simulink model "day4"  (R2017b)
settings: Solver=VariableStepAuto  StartTime=0.0  StopTime=10.0  RelTol=1e-3
undefined symbols (not defined in the file): X, Y, Z
libraries: simulink x1
settings Model: Creator=Admin  LastModifiedBy=Admin

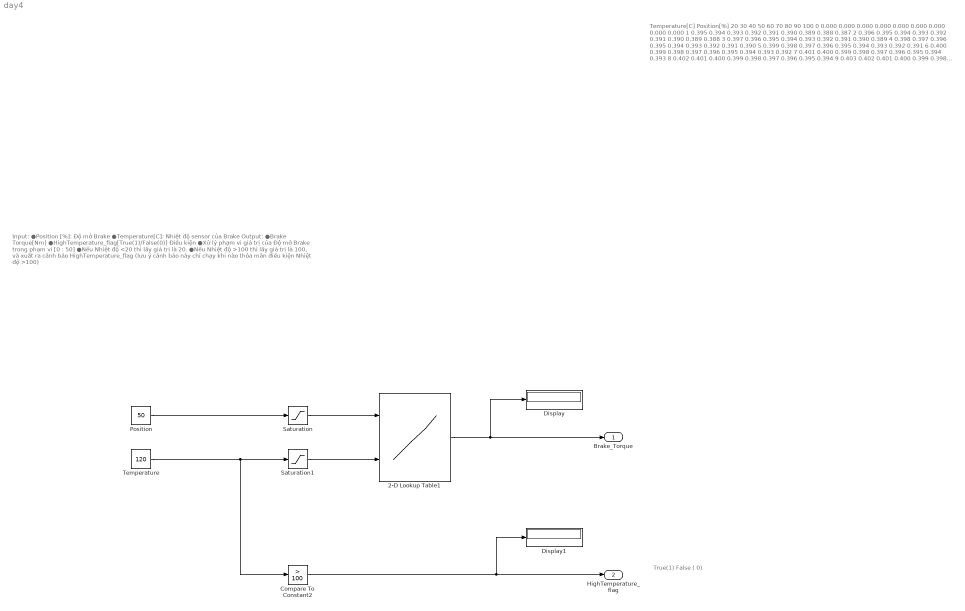
== system day4 ==
  note: Input:
      | ●Position [%]: Độ mở Brake
      | ●Temperature[C]: Nhiệt độ sensor của Brake
      | Output:
      | ●Brake Torque[Nm]
      | ●HighTemperature_flag[True(1)/False(0)]
      | Điều kiện
      | ●Xử lý phạm vi giá trị của Độ mở Brake trong phạm vi [0 : 50]
      | ●Nếu Nhiệt độ <20 thì lấy giá trị là 20.
      | ●Nếu Nhiệt độ >100 thì lấy giá trị là 100, và xuất ra cảnh báo HighTemperature_flag (lưu ý cảnh báo này chỉ chạy khi nào thỏa mãn điều kiện Nhiệt độ >100)
  note: Temperature[C]
      |
      | Position[%]
      | 20
      | 30
      | 40
      | 50
      | 60
      | 70
      | 80
      | 90
      | 100
      |
      | 0
      | 0.000
      | 0.000
      | 0.000
      | 0.000
      | 0.000
      | 0.000
      | 0.000
      | 0.000
      | 0.000
      |
      | 1
      | 0.395
      | 0.394
      | 0.393
      | 0.392
      | 0.391
      | 0.390
      | 0.389
      | 0.388
      | 0.387
      |
      | 2
      | 0.396
      | 0.395
      | 0.394
      | 0.393
      | 0.392
      | 0.391
      | 0.390
      | 0.389
      | 0.388
      |
      | 3
      | 0.397
      | 0.396
      | 0.395
      | 0.394
      | 0.393
      | 0.392
      | 0.391
      | 0.390
      | 0.389
      |
      | 4
      | 0.398
      | 0.397
      | 0.396
      | 0.395
      | 0.394
      | 0.393
      | 0.392
      | 0.391
      | 0.390
      |
      | 5
      | 0.399
      | 0.398
      | 0.397
      | 0.396
      | 0.395
      | 0.394
      | 0.393
      | 0.392
      | 0.391
      |
      | 6
      | 0.400
      | 0.399
      | 0.398
      | 0.397
      | 0.396
      | 0.395
      | 0.394
      | 0.393
      | 0.392
      |
      | 7
      | 0.401
      | 0.400
      | 0.399
      | 0.398
      | 0.397
      | 0.396
      | 0.395
      | 0.394
      | 0.393
      |
      | 8
      | 0.402
      | 0.401
      | 0.400
      | 0.399
      | 0.398
      | 0.397
      | 0.396
      | 0.395
      | 0.394
      |
      | 9
      | 0.403
      | 0.402
      | 0.401
      | 0.400
      | 0.399
      | 0.398
      | 0.397
      | 0.396
      | 0.395
      |
      | 10
      | 0.404
      | 0.403
      | 0.402
      | 0.401
      | 0.400
      | 0.399
      | 0.398
      | 0.397
      | 0.396
      |
      | 11
      | 0.405
      | 0.404
      | 0.403
      | 0.402
      | 0.401
      | 0.400
      | 0.399
      | 0.398
      | 0.397
      |
      | 12
      | 0.406
      | 0.405
      | 0.404
      | 0.403
      | 0.402
      | 0.401
      | 0.400
      | 0.399
      | 0.398
      |
      | 13
      | 0.407
      | 0.406
      | 0.405
      | 0.404
      | 0.403
      | 0.402
      | 0.401
      | 0.400
      | 0.399
      |
      | 14
      | 0.408
      | 0.407
      | 0.406
      | 0.405
      | 0.404
      | 0.403
      | 0.402
      | 0.401
      | 0.400
      |
      | 15
      | 0.409
      | 0.408
      | 0.407
      | 0.406
      | 0.405
      | 0.404
      | 0.403
      | 0.402
      | 0.401
      |
      | 16
      | 0.410
      | 0.409
      | 0.408
      | 0.407
      | 0.406
      | 0.405
      | 0.404
      | 0.403
      | 0.402
      |
      | 17
      | 0.411
      | 0.410
      | 0.409
      | 0.408
      | 0.407
      | 0.406
      | 0.405
      | 0.404
      | 0.403
      |
      | 18
      | 0.412
      | 0.411
      | 0.410
      | 0.409
      | 0.408
      | 0.407
      | 0.406
      | 0.405
      | 0.404
      |
      | 19
      | 0.413
      | 0.412
      | 0.411
      | 0.410
      | 0.409
      | 0.408
      | 0.407
      | 0.406
      | 0.405
      |
      | 20
      | 0.414
      | 0.413
      | 0.412
      | 0.411
      | 0.410
      | 0.409
      | 0.408
      | 0.407
      | 0.406
      |
      | 21
      | 0.415
      | 0.414
      | 0.413
      | 0.412
      | 0.411
      | 0.410
      | 0.409
      | 0.408
      | 0.407
      |
      | 22
      | 0.416
      | 0.415
      | 0.414
      | 0.413
      | 0.412
      | 0.411
      | 0.410
      | 0.409
      | 0.408
      |
      | 23
      | 0.417
      | 0.416
      | 0.415
      | 0.414
      | 0.413
      | 0.412
      | 0.411
      | 0.410
      | 0.409
      |
      | 24
      | 0.418
      | 0.417
      | 0.416
      | 0.415
      | 0.414
      | 0.413
      | 0.412
      | 0.411
      | 0.410
      |
      | 25
      | 0.419
      | 0.418
      | 0.417
      | 0.416
      | 0.415
      | 0.414
      | 0.413
      | 0.412
      | 0.411
      |
      | 26
      | 0.420
      | 0.419
      | 0.418
      | 0.417
      | 0.416
      | 0.415
      | 0.414
      | 0.413
      | 0.412
      |
      | 27
      | 0.421
      | 0.420
      | 0.419
      | 0.418
      | 0.417
      | 0.416
      | 0.415
      | 0.414
      | 0.413
      |
      | 28
      | 0.422
      | 0.421
      | 0.420
      | 0.419
      | 0.418
      | 0.417
      | 0.416
      | 0.415
      | 0.414
      |
      | 29
      | 0.423
      | 0.422
      | 0.421
      | 0.420
      | 0.419
      | 0.418
      | 0.417
      | 0.416
      | 0.415
      |
      | 30
      | 0.424
      | 0.423
      | 0.422
      | 0.421
      | 0.420
      | 0.419
      | 0.418
      | 0.417
      | 0.416
      |
      | 31
      | 0.425
      | 0.424
      | 0.423
      | 0.422
      | 0.421
      | 0.420
      | 0.419
      | 0.418
      | 0.417
      |
      | 32
      | 0.426
      | 0.425
      | 0.424
      | 0.423
      | 0.422
      | 0.421
      | 0.420
      | 0.419
      | 0.418
      |
      | 33
      | 0.427
      | 0.426
      | 0.425
      | 0.424
      | 0.423
      | 0.422
      | 0.421
      | 0.420
      | 0.419
      |
      | 34
      | 0.428
      | 0.427
      | 0.426
      | 0.425
      | 0.424
      | 0.423
      | 0.422
      | 0.421
      | 0.420
      |
      | 35
      | 0.429
      | 0.428
      | 0.427
      | 0.426
      | 0.425
      | 0.424
      | 0.423
      | 0.422
      | 0.421
      |
      | 36
      | 0.430
      | 0.429
      | 0.428
      | 0.427
      | 0.426
      | 0.425
      | 0.424
      | 0.423
      | 0.422
      |
      | 37
      | 0.431
      | 0.430
      | 0.429
      | 0.428
      | 0.427
      | 0.426
      | 0.425
      | 0.424
      | 0.423
      |
      | 38
      | 0.432
      | 0.431
      | 0.430
      | 0.429
      | 0.428
      | 0.427
      | 0.426
      | 0.425
      | 0.424
      |
      | 39
      | 0.433
      | 0.432
      | 0.431
      | 0.430
      | 0.429
      | 0.428
      | 0.427
      | 0.426
      | 0.425
      |
      | 40
      | 0.434
      | 0.433
      | 0.432
      | 0.431
      | 0.430
      | 0.429
      | 0.428
      | 0.427
      | 0.426
      |
      | 41
      | 0.435
      | 0.434
      | 0.433
      | 0.432
      | 0.431
      | 0.430
      | 0.429
      | 0.428
      | 0.427
      |
      | 42
      | 0.436
      | 0.435
      | 0.434
      | 0.433
      | 0.432
      | 0.431
      | 0.430
      | 0.429
      | 0.428
      |
      | 43
      | 0.437
      | 0.436
      | 0.435
      | 0.434
      | 0.433
      | 0.432
      | 0.431
      | 0.430
      | 0.429
      |
      | 44
      | 0.438
      | 0.437
      | 0.436
      | 0.435
      | 0.434
      | 0.433
      | 0.432
      | 0.431
      | 0.430
      |
      | 45
      | 0.439
      | 0.438
      | 0.437
      | 0.436
      | 0.435
      | 0.434
      | 0.433
      | 0.432
      | 0.431
      |
      | 46
      | 0.440
      | 0.439
      | 0.438
      | 0.437
      | 0.436
      | 0.435
      | 0.434
      | 0.433
      | 0.432
      |
      | 47
      | 0.441
      | 0.440
      | 0.439
      | 0.438
      | 0.437
      | 0.436
      | 0.435
      | 0.434
      | 0.433
      |
      | 48
      | 0.442
      | 0.441
      | 0.440
      | 0.439
      | 0.438
      | 0.437
      | 0.436
      | 0.435
      | 0.434
      |
      | 49
      | 0.443
      | 0.442
      | 0.441
      | 0.440
      | 0.439
      | 0.438
      | 0.437
      | 0.436
      | 0.435
      |
      | 50
      | 0.444
      | 0.443
      | 0.442
      | 0.441
      | 0.440
      | 0.439
      | 0.438
      | 0.437
      | 0.436
  note: True(1)
      | False ( 0)
  2-D Lookup Table1 : Lookup_n-D  BreakpointsForDimension1=X  BreakpointsForDimension2=Y  Table=Z  InternalRulePriority=Speed  RndMeth=Simplest  InputSameDT=on
  Compare To Constant2 : simulink/Logic and Bit Operations/Compare To Constant  relop=>  const=100  OutDataTypeStr=boolean
  Display : Display
  Display1 : Display
  Position : Constant  Description=Độ mở Brake [%]  Value=50
      settings: AttributesFormatString=%<Description>
  Saturation : Saturate  Description=[0 : 50]  UpperLimit=50  LowerLimit=0
      settings: AttributesFormatString=%<Description>
  Saturation1 : Saturate  Description=[20 : 100]  UpperLimit=100  LowerLimit=20
      settings: AttributesFormatString=%<Description>
  Temperature : Constant  Description=Nhiệt độ sensor của Brake [C]  Value=120
      settings: AttributesFormatString=%<Description>
  Brake_Torque : Outport
  HighTemperature_flag : Outport  Port=2
  wires:
  Position/1 -> Saturation/1
  Saturation/1 -> 2-D Lookup Table1/1
  2-D Lookup Table1/1 -> Display/1, Brake_Torque/1
  Compare To Constant2/1 -> HighTemperature_flag/1, Display1/1
  Temperature/1 -> Saturation1/1, Compare To Constant2/1
  Saturation1/1 -> 2-D Lookup Table1/2
